simulink model "satellite_GVE_model_sim"  (R2021a)
settings: Solver=VariableStepAuto  StartTime=0.0  StopTime=300000  RelTol=1e-3
values from neighbouring files (symbols this model uses):
  a_ini = (960e3+1019e3)/2+R_e    (= 7367700)    [Satellite_MPC3.m]
  e_ini = 0.0039866    [Satellite_MPC3.m]
  i_ini = 82.9236/180*pi()    [Satellite_MPC3.m]
  meu = G*m_e    (= 397865500000000)    [Satellite_MPC3.m]
  Ohm_ini = 272.9481/180*pi()    [Satellite_MPC3.m]
  R_e = 6378.2e3    (= 6378200)    [Satellite_MPC3.m]
  theta_ini = 0    [Satellite_MPC3.m]
  w_ini = 297.2910/180*pi()    [Satellite_MPC3.m]
settings Model: Creator=18214  LastModifiedBy=18214

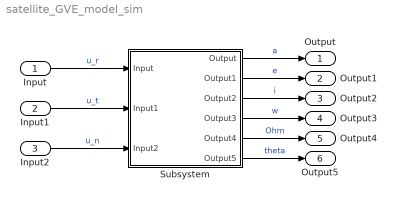
== system satellite_GVE_model_sim ==
  Input : Inport
  Input1 : Inport  Port=2
  Input2 : Inport  Port=3
  Subsystem : Subsystem
  Output : Outport
  Output1 : Outport  Port=2
  Output2 : Outport  Port=3
  Output3 : Outport  Port=4
  Output4 : Outport  Port=5
  Output5 : Outport  Port=6
  wires:
  Input/1 -> Subsystem/1(Input)  "u_r"
  Input1/1 -> Subsystem/2(Input1)  "u_t"
  Input2/1 -> Subsystem/3(Input2)  "u_n"
  Subsystem/1(Output) -> Output/1  "a"
  Subsystem/2(Output1) -> Output1/1  "e"
  Subsystem/3(Output2) -> Output2/1  "i"
  Subsystem/4(Output3) -> Output3/1  "w"
  Subsystem/5(Output4) -> Output4/1  "Ohm"
  Subsystem/6(Output5) -> Output5/1  "theta"

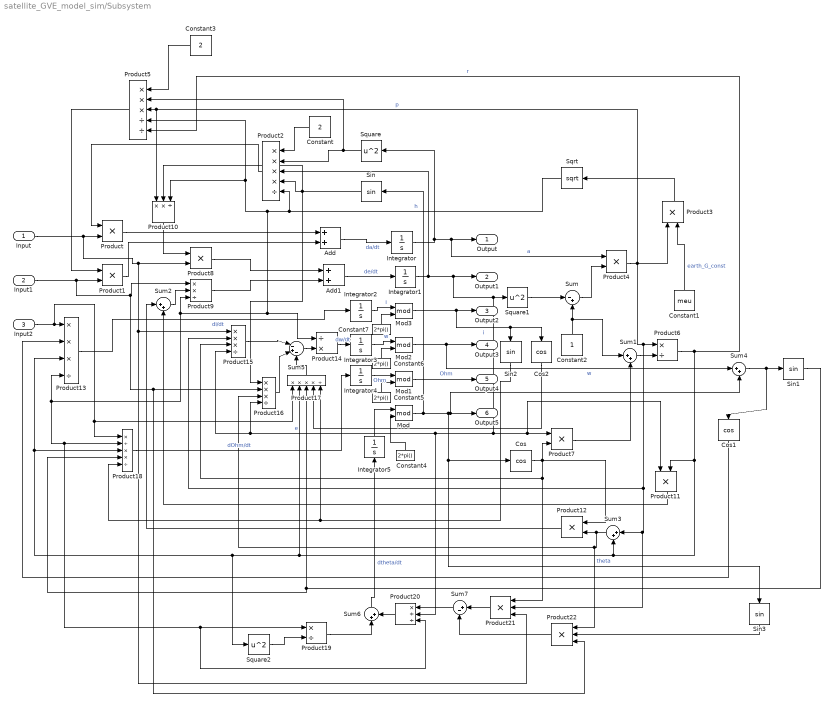
== system satellite_GVE_model_sim/Subsystem ==
  Input : Inport
  Input1 : Inport  Port=2
  Input2 : Inport  Port=3
  Add : Sum
  Add1 : Sum
  Constant : Constant  Value=2
  Constant1 : Constant  Value=meu
  Constant2 : Constant
  Constant3 : Constant  Value=2
  Constant{4..7} (4 alike) : Constant  Value=2*pi()
  Cos : Trigonometry  Operator=cos
  Cos1 : Trigonometry  Operator=cos
  Cos2 : Trigonometry  Operator=cos
  Integrator : Integrator  InitialCondition=a_ini  LimitOutput=on  LowerSaturationLimit=R_e
  Integrator1 : Integrator  InitialCondition=e_ini  LimitOutput=on  UpperSaturationLimit=1  LowerSaturationLimit=0
  Integrator2 : Integrator  InitialCondition=i_ini
  Integrator3 : Integrator  InitialCondition=w_ini
  Integrator4 : Integrator  InitialCondition=Ohm_ini
  Integrator5 : Integrator  InitialCondition=theta_ini
  Mod{,1..3} (4 alike) : Math  Operator=mod  SaturateOnIntegerOverflow=on
  Product{,1,3..4,7..8,11..12} (8 alike) : Product
  Product10 : Product  Inputs=**/
  Product13 : Product  Inputs=***/
  Product14 : Product  Inputs=/*
  Product15 : Product  Inputs=***/
  Product16 : Product  Inputs=***/
  Product17 : Product  Inputs=****/
  Product18 : Product  Inputs=*/**/
  Product19 : Product  Inputs=*/
  Product2 : Product  Inputs=****/
  Product20 : Product  Inputs=*//
  Product21 : Product  Inputs=***
  Product22 : Product  Inputs=***
  Product5 : Product  Inputs=***//
  Product6 : Product  Inputs=*/
  Product9 : Product  Inputs=**/
  Sin{,1..3} (4 alike) : Trigonometry
  Sqrt : Sqrt  SaturateOnIntegerOverflow=on
  Square : Math  Operator=square  SaturateOnIntegerOverflow=on
  Square1 : Math  Operator=square  SaturateOnIntegerOverflow=on
  Square2 : Math  Operator=square  SaturateOnIntegerOverflow=on
  Sum : Sum  Inputs=|-+
  Sum{1..4,6} (5 alike) : Sum  Inputs=|++
  Sum5 : Sum  Inputs=|-+-
  Sum7 : Sum  Inputs=|+-
  Output : Outport
  Output1 : Outport  Port=2
  Output2 : Outport  Port=3
  Output3 : Outport  Port=4
  Output4 : Outport  Port=5
  Output5 : Outport  Port=6
  wires:
  Integrator/1 -> Square/1, Output/1, Product4/1  "a"
  Square2/1 -> Product19/2
  Product2/1 -> Product/1
  Mod/1 -> Sin/1, Output5/1, Sum4/2, Cos/1, Sin3/1  "theta"
  Sin1/1 -> Product18/4, Product17/3
  Product21/1 -> Sum7/1
  Sum5/1 -> Product14/2
  Cos/1 -> Product21/1, Product15/3, Product12/1, Product7/2
  Product4/1 -> Product15/2, Product21/2, Sum3/1, Product6/1, Product10/1, Product5/3, Product3/1  "p"
  Cos2/1 -> Product17/4
  Sin/1 -> Product16/1, Product10/2, Product2/4
  Sqrt/1 -> Product10/3, Product5/4, Product13/4, Product20/3, Product19/1, Product18/2, Product9/3, Product14/1, Product2/5  "h"
  Product12/1 -> Sum2/1
  Sum/1 -> Product4/2
  Sum3/1 -> Product22/1, Product16/3, Product12/2
  Sum7/1 -> Product20/1
  Product1/1 -> Add/2
  Product22/1 -> Sum7/2
  Input/1 -> Product21/3, Product15/1, Product8/2, Product/2
  Product7/1 -> Sum1/2
  Product5/1 -> Product1/1
  Sin3/1 -> Product22/2
  Product15/1 -> Sum5/1
  Integrator1/1 -> Product2/3, Output1/1, Square1/1, Product7/1, Product11/1, Product20/2, Product16/4, Product15/4  "e"
  Sum1/1 -> Product6/2
  Cos1/1 -> Product13/2
  Product19/1 -> Sum6/1
  Product8/1 -> Add1/1
  Product6/1 -> Product5/5, Square2/1, Product13/3, Product18/3, Product17/2, Sum3/2, Product11/2  "r"
  Constant2/1 -> Sum/2, Sum1/1
  Square/1 -> Product5/2, Product2/2
  Product11/1 -> Sum2/2
  Product/1 -> Add/1
  Mod3/1 -> Output2/1, Sin2/1, Cos2/1  "i"
  Sin2/1 -> Product18/5, Product17/5
  Product17/1 -> Sum5/3
  Product16/1 -> Sum5/2
  Sum6/1 -> Integrator5/1  "dtheta/dt"
  Product10/1 -> Product8/1
  Product9/1 -> Add1/2
  Sum4/1 -> Sin1/1, Cos1/1
  Product20/1 -> Sum6/2
  Mod2/1 -> Output3/1, Sum4/1  "w"
  Input1/1 -> Product22/3, Product16/2, Product9/1, Product1/2
  Constant/1 -> Product2/1
  Sum2/1 -> Product9/2
  Product14/1 -> Integrator3/1  "dw/dt"
  Square1/1 -> Sum/1
  Input2/1 -> Product18/1, Product17/1, Product13/1
  Product13/1 -> Integrator2/1  "di/dt"
  Add/1 -> Integrator/1  "da/dt"
  Constant1/1 -> Product3/2  "earth_G_const"
  Mod1/1 -> Output4/1  "Ohm"
  Product18/1 -> Integrator4/1  "dOhm/dt"
  Add1/1 -> Integrator1/1  "de/dt"
  Constant3/1 -> Product5/1
  Product3/1 -> Sqrt/1
  Integrator5/1 -> Mod/1
  Constant4/1 -> Mod/2
  Constant5/1 -> Mod1/2
  Integrator4/1 -> Mod1/1  "Ohm"
  Constant6/1 -> Mod2/2
  Integrator3/1 -> Mod2/1  "w"
  Constant7/1 -> Mod3/2
  Integrator2/1 -> Mod3/1  "i"
